simulink model "mass2"  (R2022a)
settings: Solver=VariableStepAuto  StartTime=0.0  StopTime=5  MaxStep=0.025  RelTol=1e-3  AbsTol=1e-3
PreLoadFcn:
  | m = 3.600; %Kg
  | k = 400; %N/m
  | b = 10; %N/(m/s)
  | x0 = 1; %m
Description:
  | Sistema massa mola amortecedor
settings Model: Creator=kawha  LastModifiedBy=kawha

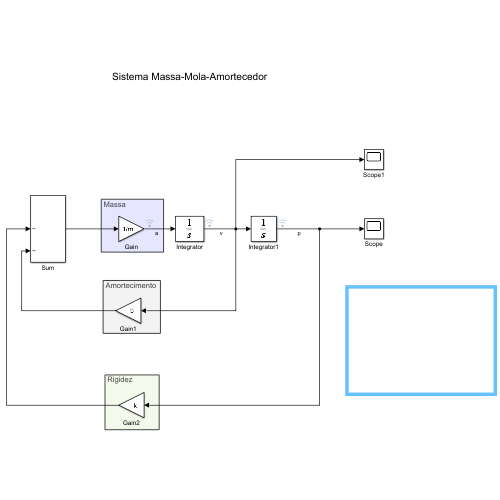
[thumbnail: Simulink's stored preview of the top-level diagram]
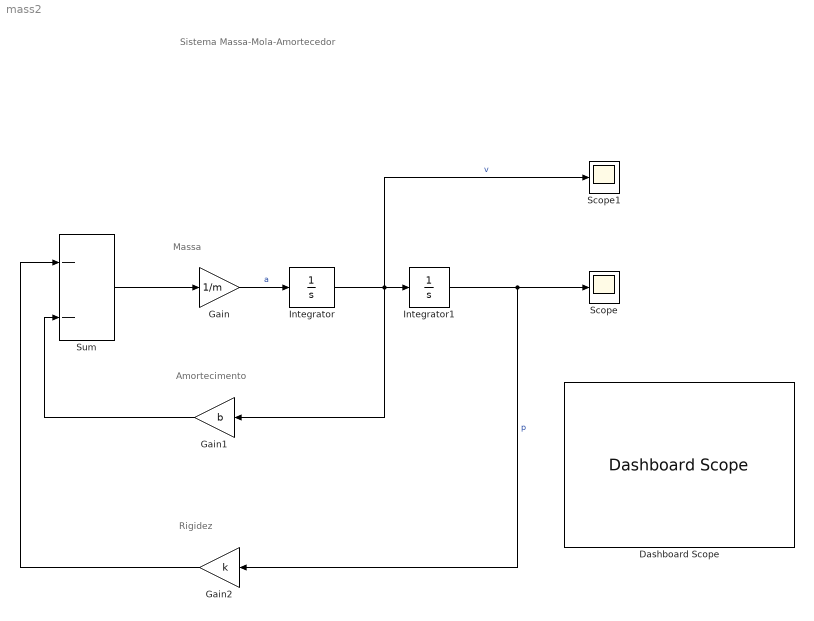
== system mass2 ==
  note: Rigidez
  note: Amortecimento
  note: Massa
  note: Sistema Massa-Mola-Amortecedor
  Dashboard Scope : DashboardScope
  Gain : Gain  Gain=1/m  ParamDataTypeStr=Inherit: Same as input
  Gain1 : Gain  Gain=b  ParamDataTypeStr=Inherit: Same as input
  Gain2 : Gain  Gain=k  ParamDataTypeStr=Inherit: Same as input
  Integrator : Integrator
  Integrator1 : Integrator  InitialCondition=1
  Scope : Scope
  Scope1 : Scope
  Sum : Sum  Inputs=|--
  wires:
  Sum/1 -> Gain/1
  Gain/1 -> Integrator/1  "a"
  Integrator/1 -> Scope1/1, Integrator1/1, Gain1/1  "v"
  Gain1/1 -> Sum/2
  Integrator1/1 -> Scope/1, Gain2/1  "p"
  Gain2/1 -> Sum/1
